simulink model "PID_wPlant"  (R2018b)
settings: Solver=FixedStepAuto  StartTime=0.0  StopTime=10  FixedStep=0.01  RelTol=1e-3
InitFcn:
  | PID_wPlant_Init
values from neighbouring files (symbols this model uses):
  Pos = 1    [PID_wPlant_Init.m]
libraries: Controller_Lib x2
settings Model: Creator=turker.erbasi  LastModifiedBy=turker.erbasi

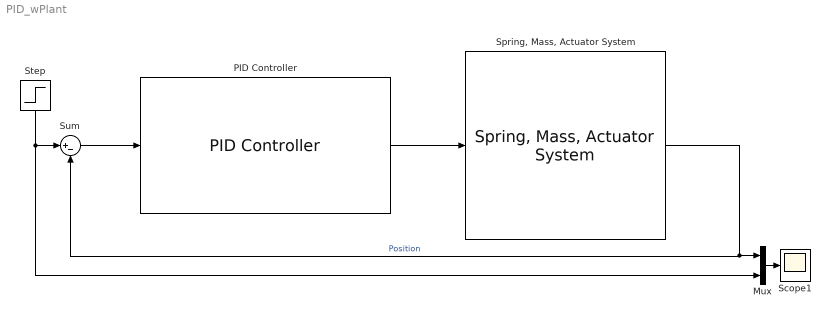
== system PID_wPlant ==
  Mux : Mux  Inputs=2
  PID Controller : Controller_Lib/PID Controller  SystemSampleTime=-1
      link override K_d: Gain=K_d
      link override K_i: Gain=K_i
      link override K_p: Gain=K_p
  Scope1 : Scope
  "Spring, Mass, Actuator System" : Controller_Lib/Spring, Mass, Actuator System  SystemSampleTime=-1
  Step : Step  After=Pos  SampleTime=0
  Sum : Sum  Inputs=|+-
  wires:
  PID Controller/1 -> "Spring, Mass, Actuator System"/1
  Sum/1 -> PID Controller/1
  Step/1 -> Sum/1, Mux/2
  "Spring, Mass, Actuator System"/1 -> Sum/2, Mux/1  "Position"
  Mux/1 -> Scope1/1
